simulink model "quad_animation"  (R2018b)
settings: Solver=FixedStepDiscrete  StartTime=0.0  StopTime=10000  FixedStep=.1  RelTol=1e-3  EnableMultiTasking=on
undefined symbols (not defined in the file or in its folder): drawQuad
libraries: simulink x6
settings Model: Creator=beard  LastModifiedBy=erics
settings DataIOCC: LimitDataPoints=on  SaveFormat=Array  SignalLoggingSaveFormat=ModelDataLogs
settings OptimizationCC: ExpressionDepthLimit=2147483647  InitFltsAndDblsToZero=on  LifeSpan=inf
settings DebuggingCC: UnderspecifiedInitializationDetection=Classic  MergeDetectMultiDrivingBlocksExec=none  SolverPrmCheckMsg=warning  FcnCallInpInsideContextMsg=warning  StateNameClashWarn=warning  SFUnexpectedBacktrackingDiag=warning  SFNoUnconditionalDefaultTransitionDiag=warning  SFExecutionAtInitializationDiag=none
settings HardwareCC: ProdBitPerPointer=32  ProdBitPerSizeT=32  ProdBitPerPtrDiffT=32  ProdLargestAtomicFloat=None  ProdIntDivRoundTo=Undefined  ProdEndianess=Unspecified  ProdWordSize=32  ProdHWDeviceType=32-bit Generic
settings ModelReferenceCC: PropagateSignalLabelsOutOfModel=off
settings SFSimCC: SimUseLocalCustomCode=off
settings RTWCC: RTWUseLocalCustomCode=off
settings CodeAppCC: StateflowObjectComments=on
settings GRTTargetCC: TargetLangStandard=C89/C90 (ANSI)  GeneratePreprocessorConditionals=Disable all  CombineOutputUpdateFcns=off  GRTInterface=on
settings ConfigComp: CovMetricSettings=dw  CovHtmlReporting=on  CovSaveCumulativeToWorkspaceVar=on  CovSaveSingleToWorkspaceVar=on  CovExternalEMLEnable=off  CovSFcnEnable=off

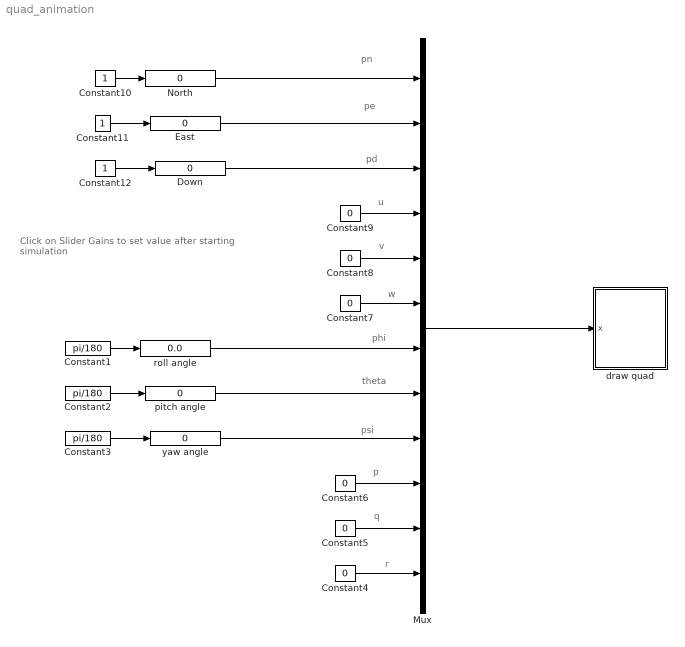
== system quad_animation ==
  note: pn
  note: pe
  note: pd
  note: phi
  note: theta
  note: psi
  note: p
  note: q
  note: r
  note: u
  note: v
  note: w
  note: Click on Slider Gains to set value
      | after starting simulation
  Constant1 : Constant  Value=pi/180
  Constant10 : Constant
  Constant11 : Constant
  Constant12 : Constant
  Constant2 : Constant  Value=pi/180
  Constant3 : Constant  Value=pi/180
  Constant{4..9} (6 alike) : Constant  Value=0
  Down : simulink/Math Operations/Slider Gain  gain=0  low=-10  high=10
  East : simulink/Math Operations/Slider Gain  gain=0  low=-10  high=10
  Mux : Mux  Inputs=12
  North : simulink/Math Operations/Slider Gain  gain=0  low=-10  high=10
  draw quad : Subsystem
      mask init:
      | P.courselength = 11;
      | P.coursewidth = 6;
      |     %6ft columns plus four feet of head room
      | P.courseheight = 10;
      | 
      | % quadrotor starting point at 3 ft high and 3 ft in front of the pillars 
      | P.zstart = 0;
      | P.xstart = 0;
      | P.ystart = 0;
      | 
      | % quadrotor dimentions
      |     %2 inches from the center
      | P.boxlength = 1/6;
      | P.boxwidth = P.boxlength;
      |     %4.5 inches from the bottom to the top
      | P.boxheight = 0.375;
      |     %6 inches from box to motor
      | P.armlength = 0.5;
      |     %1/8 inch from center to the side of a rod
      | P.armwidth = 1/96;
      |     %1/4 inch from the top of the box
      | P.armposition = 1/48;
      |     %25*(2)^(1/2)/2 inches from center to perimeter along x and y axis
      | P.perimeter = 1.47;
      |     %perimeter has 3/16 inch width
      | P.periwidth = 1/64;
      | 
      | % pillar dimentions
      |     %6 ft high
      | P.pillarheight = 6;
      |     %5 ft offset;
      | P.pillarposition = 5; 
      |     %5 in radius
      | P.pillarradius = 0.417;
      |     %The adjustment for the none circular pillar
      | P.pillaradd = 0.167;
      |     %The height of each strip on color
      | P.pillarc1 = 0.833; 
      | P.pillarc2 = 0.5;
      mask Display: image(imread('tv.jpg'))
  pitch angle : simulink/Math Operations/Slider Gain  gain=0  low=-180  high=180
  roll angle : simulink/Math Operations/Slider Gain  gain=0.0  low=-180  high=180
  "yaw angle " : simulink/Math Operations/Slider Gain  gain=0  low=-180  high=180
  wires:
  roll angle/1 -> Mux/7
  Constant1/1 -> roll angle/1
  pitch angle/1 -> Mux/8
  Constant2/1 -> pitch angle/1
  "yaw angle "/1 -> Mux/9
  Constant3/1 -> "yaw angle "/1
  Constant4/1 -> Mux/12
  Constant5/1 -> Mux/11
  Constant6/1 -> Mux/10
  Constant7/1 -> Mux/6
  Constant8/1 -> Mux/5
  Constant9/1 -> Mux/4
  North/1 -> Mux/1
  Constant10/1 -> North/1
  East/1 -> Mux/2
  Constant11/1 -> East/1
  Down/1 -> Mux/3
  Constant12/1 -> Down/1
  Mux/1 -> draw quad/1(x)

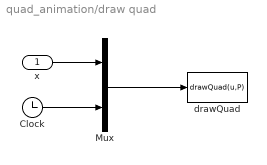
== system quad_animation/draw quad ==
  x : Inport
  Clock : Clock
  Mux : Mux  Inputs=2
  drawQuad : MATLABFcn  MATLABFcn=drawQuad(u,P)  OutputDimensions=0  SampleTime=0.1
  wires:
  Mux/1 -> drawQuad/1
  x/1 -> Mux/1
  Clock/1 -> Mux/2
